simulink model "LateralControllerDIY"  (R2021a)
settings: Solver=VariableStepAuto  StartTime=0.0  StopTime=20  RelTol=1e-3
values from neighbouring files (symbols this model uses):
  ks = 0    [controller_setup.m]    (also in test.m)
  PredictionHorizon = 60    [controller_setup.m]
  Ts = 0.05    [controller_setup.m]    (also in test.m = 0.1)
  Vx = 15    [controller_setup.m]    (also in test.m)
libraries: simulink_extras x3, mpclib x1
(part 1 of 2)
settings Model: Creator=chnwa  LastModifiedBy=chnwa

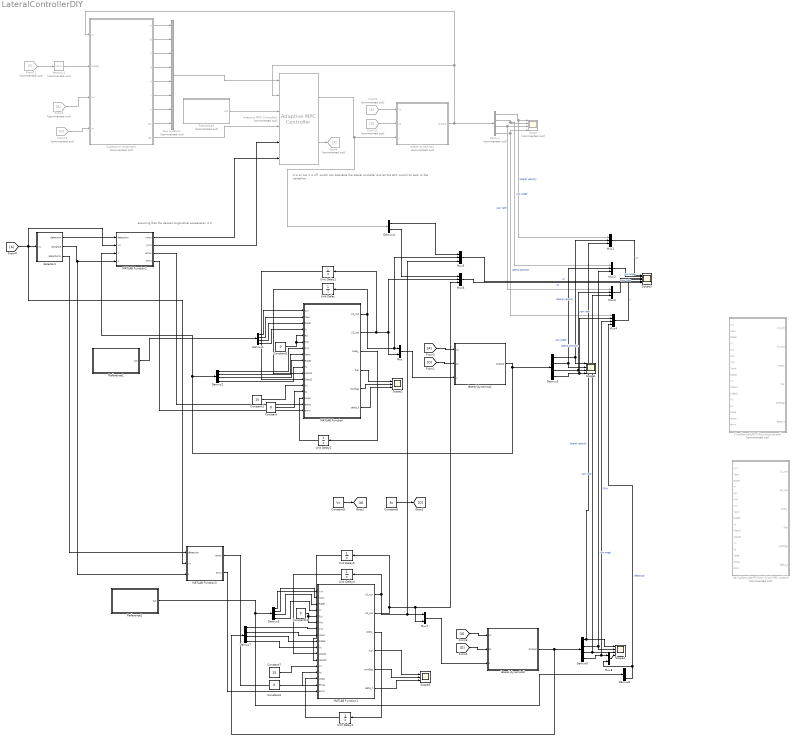
== system LateralControllerDIY ==
  note: assuming that the desired longitudinal acceleration is 0
  note: 0 is on but 1 is off. switch can disenable the lateral controller and let the ACC control its back to the centerline
  Adaptive MPC Controller1 : mpclib/Adaptive MPC Controller  Commented=on  SCDEnableBlockLinearizationSpecification=on  mpcobj=mpc007  enable_value=0  updateMPCinCallerWorkspace=on  md_inport=on  mv_inport=off  uref_inport=off  return_cost=off  return_mvseq=on  return_qpstatus=off  return_xseq=off  return_state=off  return_ovseq=off  state_inport=off  isltv_plant=on  umin_inport=off  umax_inport=off  ymin_inport=on  ymax_inport=on  cc_inport=off  ywt_inport=off  uwt_inport=off  duwt_inport=off  rhoeps_inport=off  pm_inport=off  MaximumP=10  HorizonChoice=FixedHorizon  BlockDataType=double  SampleTimeInherited=off  switch_inport=off
  Bus Creator1 : BusCreator  Commented=on  Inputs=8
  Constant{,2,4,10} (4 alike) : Constant  Value=0
  Constant1 : Constant  Value=15
  Constant5 : Constant  Value=Vx
  Constant6 : Constant  Value=ks
  Constant7 : Constant  Value=15
  Demux : Demux  Commented=on
  Demux{1..3,5..8} (7 alike) : Demux
  Demux4 : Demux  Outputs=2
  FixedSampleMPC(Non-Augmented) : MATLAB Function  Commented=on  TreatAsAtomicUnit=on
  From11 : From  Commented=on  GotoTag=F
  From12 : From  Commented=on  GotoTag=D
  From13 : From  Commented=on  GotoTag=D
  From2 : From  Commented=on
  From8 : From  Commented=on
  Goto6 : Goto  Commented=on  GotoTag=F
  MATLAB Function : MATLAB Function  TreatAsAtomicUnit=on
  MATLAB Function1 : MATLAB Function  TreatAsAtomicUnit=on
  MATLAB Function2 : MATLAB Function  TreatAsAtomicUnit=on
  MATLAB Function3 : MATLAB Function  TreatAsAtomicUnit=on
  Memory1 : Memory  Commented=on
  Mux : Mux  Inputs=2
  Mux{1..3,5..6} (5 alike) : Mux  Inputs=3
  Mux4 : Mux
  Mux7 : Mux  Inputs=2
  Mux8 : Mux  Inputs=2
  Reference1 : Subsystem  AncestorBlock=Meldas_library/Reference
  Reference2 : Subsystem  AncestorBlock=Meldas_library/Reference
  Reference3 : Subsystem  Commented=on  AncestorBlock=Meldas_library/Reference
  Scope : Scope  Commented=on  NumInputPorts=4
  Scope1 : Scope  NumInputPorts=4
  Scope2 : Scope  NumInputPorts=3
  Scope3 : Scope  NumInputPorts=6
  Scope4 : Scope  NumInputPorts=4
  Scope5 : Scope  NumInputPorts=3
  Successive Linearizer1 : MATLAB Function  Commented=on  TreatAsAtomicUnit=on
  Unit Delay{,1,4..5} (4 alike) : UnitDelay  SampleTime=-1  HasFrameUpgradeWarning=on
  Unit Delay2 : UnitDelay  InitialCondition=zeros(61,2)  SampleTime=-1  HasFrameUpgradeWarning=on
  Unit Delay3 : UnitDelay  InitialCondition=zeros(71,2)  SampleTime=-1  HasFrameUpgradeWarning=on
  VaringSampleMPC(Non-fixed MPC added) : MATLAB Function  Commented=on  TreatAsAtomicUnit=on
  detector1 : Subsystem
  lateral dynamics1 : Subsystem
  lateral dynamics2 : Subsystem  Commented=on
  lateral dynamics3 : Subsystem
  wires:
  Adaptive MPC Controller1/1 -> Demux4/1, lateral dynamics2/3(u)
  Constant6/1 -> [D]
  MATLAB Function2/2(ymin) -> Adaptive MPC Controller1/5
  Constant5/1 -> [A]
  Memory1/1 -> Successive Linearizer1/2(moves)
  From2/1 -> Successive Linearizer1/3(Vx)
  From8/1 -> lateral dynamics2/1(Vx)
  lateral dynamics2/1(Output) -> Demux/1, Successive Linearizer1/1(xk), Adaptive MPC Controller1/2
  From12/1 -> lateral dynamics2/2(ks)
  Successive Linearizer1/3(C) -> Bus Creator1/3
  Successive Linearizer1/5(U) -> Bus Creator1/5
  Successive Linearizer1/4(D) -> Bus Creator1/4
  Successive Linearizer1/2(B) -> Bus Creator1/2
  Bus Creator1/1 -> Adaptive MPC Controller1/1
  Successive Linearizer1/1(A) -> Bus Creator1/1
  Reference3/1(out) -> Adaptive MPC Controller1/3
  From13/1 -> Successive Linearizer1/4(ks)
  Successive Linearizer1/6(Y) -> Bus Creator1/6
  Successive Linearizer1/7(X) -> Bus Creator1/7
  detector1/2(distance) -> MATLAB Function3/3(s), MATLAB Function2/4(s)
  From11/1 -> Memory1/1
  MATLAB Function2/1(ymax) -> Adaptive MPC Controller1/6
  [A] -> MATLAB Function3/2(Vx), MATLAB Function2/2(Vx), detector1/1(Vx)
  Successive Linearizer1/8(DX) -> Bus Creator1/8
  Adaptive MPC Controller1/2 -> Goto6/1
  Successive Linearizer1/9(DK) -> Adaptive MPC Controller1/4
  Demux/1 -> Mux1/1, Scope/1  "lateral velocity"
  Demux/2 -> Mux2/1, Scope/2  "yaw angel"
  Demux/3 -> Mux3/1, Scope/3  "yaw rate"
  Demux/4 -> Mux4/1, Scope/4  "lateral position"
  MATLAB Function/1(U1_out) -> Mux5/2, Mux/1, Unit Delay/1
  Unit Delay/1 -> MATLAB Function/11(Ulast1)
  MATLAB Function/2(U2_out) -> Mux6/2, Mux/2, Unit Delay1/1
  Unit Delay1/1 -> MATLAB Function/12(Ulast2)
  MATLAB Function/3(Useq_) -> Unit Delay2/1
  Unit Delay2/1 -> MATLAB Function/15(Useq)
  Constant/1 -> MATLAB Function/14(ks)
  Constant1/1 -> MATLAB Function/13(Vx)
  Reference1/1(out) -> Demux1/1
  Demux1/1 -> MATLAB Function/1(Vyr)
  Demux1/2 -> MATLAB Function/2(Yawr)
  Demux1/3 -> MATLAB Function/3(Rater)
  Demux1/4 -> MATLAB Function/4(Yr)
  Constant2/1 -> MATLAB Function/5(Fyr), MATLAB Function/6(Mxr)
  [A] -> lateral dynamics1/1(Vx)
  [D] -> lateral dynamics1/2(ks)
  Mux/1 -> lateral dynamics1/3(u)
  Demux2/1 -> MATLAB Function/7(Vyc)
  Demux2/2 -> MATLAB Function/8(Yawc)
  Demux2/3 -> MATLAB Function/9(Ratec)
  Demux2/4 -> MATLAB Function/10(Yc)
  Demux3/2 -> Scope1/2, Mux2/2  "yaw angel"
  Demux3/3 -> Mux3/2, Scope1/3  "yaw rate"
  Demux3/1 -> Scope1/1, Mux1/2  "lateral velocity"
  lateral dynamics1/1(Output) -> MATLAB Function2/3(x), Demux2/1, Demux3/1
  Demux3/4 -> Mux4/2, Scope1/4  "lateral position"
  MATLAB Function/4(fval) -> Scope2/1
  MATLAB Function/5(exitflag) -> Scope2/2
  MATLAB Function/6(delta_t) -> Scope2/3
  Mux1/1 -> Scope3/1  "Vy"
  Mux2/1 -> Scope3/2  "yaw angle"
  Mux3/1 -> Scope3/3  "yaw rate"
  Mux4/1 -> Scope3/4  "Y"
  Demux4/1 -> Mux5/1
  Demux4/2 -> Mux6/1
  Mux5/1 -> Scope3/5  "u1"
  Mux6/1 -> Scope3/6  "u2"
  MATLAB Function1/1(U1_out) -> Unit Delay4/1, Mux5/3, Mux7/1
  Unit Delay4/1 -> MATLAB Function1/11(Ulast1)
  MATLAB Function1/2(U2_out) -> Mux6/3, Mux7/2, Unit Delay5/1
  Unit Delay5/1 -> MATLAB Function1/12(Ulast2)
  MATLAB Function1/3(Useq_) -> Unit Delay3/1
  Unit Delay3/1 -> MATLAB Function1/15(Useq)
  Constant7/1 -> MATLAB Function1/13(Vx)
  Constant4/1 -> MATLAB Function1/14(ks)
  Demux5/4 -> MATLAB Function1/4(Yr)
  Reference2/1(out) -> Demux8/1, Demux5/1
  Demux5/3 -> MATLAB Function1/3(Rater)
  Demux5/2 -> MATLAB Function1/2(Yawr)
  Demux5/1 -> MATLAB Function1/1(Vyr)
  Constant10/1 -> MATLAB Function1/5(Fyr), MATLAB Function1/6(Mxr)
  [A] -> lateral dynamics3/1(Vx)
  [D] -> lateral dynamics3/2(ks)
  Mux7/1 -> lateral dynamics3/3(u)
  Demux6/2 -> Mux2/3, Scope4/2  "yaw angel"
  Demux6/3 -> Scope4/3, Mux3/3  "yaw rate"
  Demux6/1 -> Mux1/3, Scope4/1  "lateral velocity"
  lateral dynamics3/1(Output) -> Demux7/1, Demux6/1
  Demux6/4 -> Mux4/3, Mux8/1  "FOH"
  Demux7/1 -> MATLAB Function1/7(Vyc)
  Demux7/2 -> MATLAB Function1/8(Yawc)
  Demux7/3 -> MATLAB Function1/9(Ratec)
  Demux7/4 -> MATLAB Function1/10(Yc)
  MATLAB Function1/4(fval) -> Scope5/1
  MATLAB Function1/6(delta_t) -> Scope5/3
  MATLAB Function1/5(exitflag) -> Scope5/2
  MATLAB Function2/3(emax) -> MATLAB Function/16(emax)
  MATLAB Function2/4(emin) -> MATLAB Function/17(emin)
  detector1/1(detection) -> MATLAB Function2/1(detection)
  Demux8/4 -> Mux4/4, Mux8/2  "reference"
  Mux8/1 -> Scope4/4
  detector1/3(detection1) -> MATLAB Function3/1(detection)
  MATLAB Function3/1(emax) -> MATLAB Function1/16(emax)
  MATLAB Function3/2(emin) -> MATLAB Function1/17(emin)

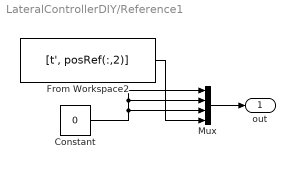
== system LateralControllerDIY/Reference1 ==
  Constant : Constant  Value=0
  From Workspace2 : FromWorkspace  VariableName=[t', posRef(:,2)]  SampleTime=0.1
  Mux : Mux
  out : Outport  VectorParamsAs1DForOutWhenUnconnected=off
  wires:
  From Workspace2/1 -> Mux/4
  Constant/1 -> Mux/3, Mux/2, Mux/1
  Mux/1 -> out/1

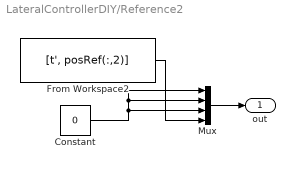
== system LateralControllerDIY/Reference2 ==
  Constant : Constant  Value=0
  From Workspace2 : FromWorkspace  VariableName=[t', posRef(:,2)]  SampleTime=0.1
  Mux : Mux
  out : Outport  VectorParamsAs1DForOutWhenUnconnected=off
  wires:
  From Workspace2/1 -> Mux/4
  Constant/1 -> Mux/3, Mux/2, Mux/1
  Mux/1 -> out/1

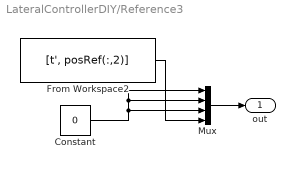
== system LateralControllerDIY/Reference3 ==
  Constant : Constant  Value=0
  From Workspace2 : FromWorkspace  VariableName=[t', posRef(:,2)]  SampleTime=0.1
  Mux : Mux
  out : Outport  VectorParamsAs1DForOutWhenUnconnected=off
  wires:
  From Workspace2/1 -> Mux/4
  Constant/1 -> Mux/3, Mux/2, Mux/1
  Mux/1 -> out/1

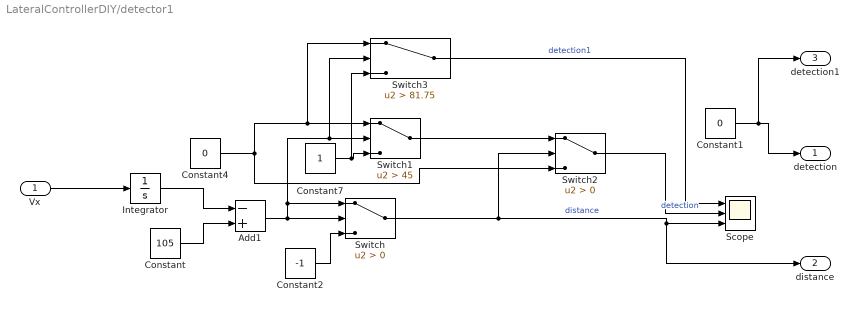
== system LateralControllerDIY/detector1 ==
  Vx : Inport
  Add1 : Sum  Inputs=-+
  Constant : Constant  Value=105
  Constant1 : Constant  Value=0
  Constant2 : Constant  Value=-1
  Constant4 : Constant  Value=0
  Constant7 : Constant
  Integrator : Integrator
  Scope : Scope  NumInputPorts=3
  Switch : Switch  Criteria=u2 > Threshold
  Switch1 : Switch  Criteria=u2 > Threshold  Threshold=45
  Switch2 : Switch  Criteria=u2 > Threshold
  Switch3 : Switch  Criteria=u2 > Threshold  Threshold=81.75
  detection : Outport
  distance : Outport  Port=2
  detection1 : Outport  Port=3
  wires:
  Constant2/1 -> Switch/3
  Constant4/1 -> Switch2/3, Switch3/1, Switch1/1
  Vx/1 -> Integrator/1
  Integrator/1 -> Add1/1
  Switch/1 -> Switch2/2, distance/1, Scope/3  "distance"
  Constant7/1 -> Switch3/3, Switch1/3
  Add1/1 -> Switch3/2, Switch1/2, Switch/1, Switch/2
  Switch1/1 -> Switch2/1
  Constant/1 -> Add1/2
  Switch2/1 -> Scope/2  "detection"
  Switch3/1 -> Scope/1  "detection1"
  Constant1/1 -> detection1/1, detection/1

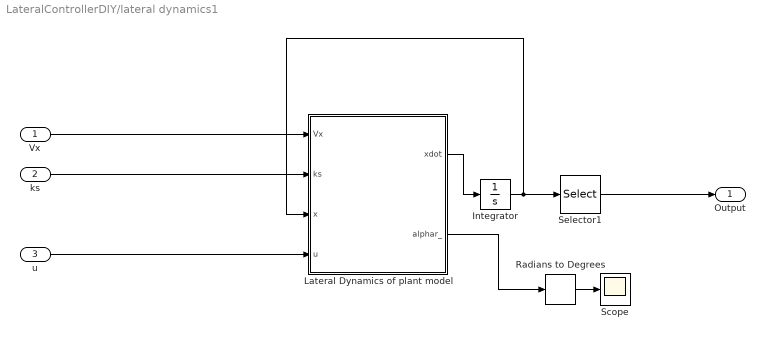
== system LateralControllerDIY/lateral dynamics1 ==
  Vx : Inport
  ks : Inport  Port=2
  u : Inport  Port=3
  Integrator : Integrator
  Lateral Dynamics of plant model : MATLAB Function  TreatAsAtomicUnit=on
  Radians to Degrees : simulink_extras/Transformations/Radians to Degrees
  Scope : Scope
  Selector1 : Selector  InputPortWidth=4  IndexOptions=Index vector (dialog)  Indices=[1 2 3 4]  OutputSizes=1
  Output : Outport
  wires:
  u/1 -> Lateral Dynamics of plant model/4(u)
  Lateral Dynamics of plant model/1(xdot) -> Integrator/1
  Integrator/1 -> Selector1/1, Lateral Dynamics of plant model/3(x)
  Selector1/1 -> Output/1
  ks/1 -> Lateral Dynamics of plant model/2(ks)
  Vx/1 -> Lateral Dynamics of plant model/1(Vx)
  Lateral Dynamics of plant model/2(alphar_) -> Radians to Degrees/1
  Radians to Degrees/1 -> Scope/1

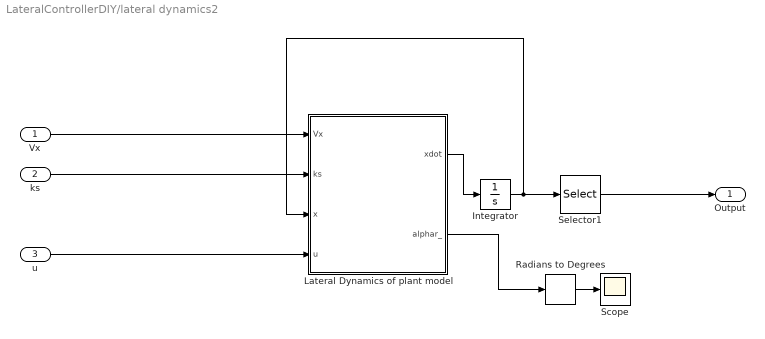
== system LateralControllerDIY/lateral dynamics2 ==
  Vx : Inport
  ks : Inport  Port=2
  u : Inport  Port=3
  Integrator : Integrator
  Lateral Dynamics of plant model : MATLAB Function  TreatAsAtomicUnit=on
  Radians to Degrees : simulink_extras/Transformations/Radians to Degrees
  Scope : Scope
  Selector1 : Selector  InputPortWidth=4  IndexOptions=Index vector (dialog)  Indices=[1 2 3 4]  OutputSizes=1
  Output : Outport
  wires:
  u/1 -> Lateral Dynamics of plant model/4(u)
  Lateral Dynamics of plant model/1(xdot) -> Integrator/1
  Integrator/1 -> Selector1/1, Lateral Dynamics of plant model/3(x)
  Selector1/1 -> Output/1
  ks/1 -> Lateral Dynamics of plant model/2(ks)
  Vx/1 -> Lateral Dynamics of plant model/1(Vx)
  Lateral Dynamics of plant model/2(alphar_) -> Radians to Degrees/1
  Radians to Degrees/1 -> Scope/1

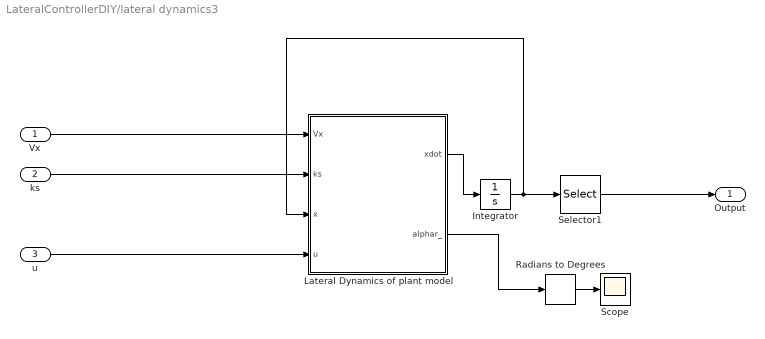
== system LateralControllerDIY/lateral dynamics3 ==
  Vx : Inport
  ks : Inport  Port=2
  u : Inport  Port=3
  Integrator : Integrator
  Lateral Dynamics of plant model : MATLAB Function  TreatAsAtomicUnit=on
  Radians to Degrees : simulink_extras/Transformations/Radians to Degrees
  Scope : Scope
  Selector1 : Selector  InputPortWidth=4  IndexOptions=Index vector (dialog)  Indices=[1 2 3 4]  OutputSizes=1
  Output : Outport
  wires:
  u/1 -> Lateral Dynamics of plant model/4(u)
  Lateral Dynamics of plant model/1(xdot) -> Integrator/1
  Integrator/1 -> Selector1/1, Lateral Dynamics of plant model/3(x)
  Selector1/1 -> Output/1
  ks/1 -> Lateral Dynamics of plant model/2(ks)
  Vx/1 -> Lateral Dynamics of plant model/1(Vx)
  Lateral Dynamics of plant model/2(alphar_) -> Radians to Degrees/1
  Radians to Degrees/1 -> Scope/1

== matlab function LateralControllerDIY/Successive Linearizer1 ==
  data: A output size=[4,4,PredictionHorizon+1]; xk input size=[4,1]; moves input; B output size=[4,6,PredictionHorizon+1]; C output size=[4,4,PredictionHorizon+1]; D output size=[4,6,PredictionHorizon+1]; U output size=[6,1,PredictionHorizon+1]; Y output size=[4,1,PredictionHorizon+1]; X output size=[4,1,PredictionHorizon+1]; DX output size=[4,1,PredictionHorizon+1]; Vx input size=1; ks input; PredictionHorizon parameter size=1; DK output; Ts parameter size=1
function [A,B,C,D,U,Y,X,DX,DK] = fcn(xk,moves,Vx,ks, PredictionHorizon, Ts)
%sucessive updates the LTI plant model required by adaptive MPC controller
% LTV MPC requires p+1 linearizations from k to k+p
Steps = PredictionHorizon + 1; % having the number of Steps models
% Initialize outputs
A = zeros(4,4,Steps);
B = zeros(4,6,Steps);
C = zeros(4,4,Steps);
D = zeros(4,6,Steps);
U = zeros(6,1,Steps);
Y = zeros(4,1,Steps);
X = zeros(4,1,Steps);
DX = zeros(4,1,Steps);
DK = zeros(Steps,4); % the constant matrix in the model considered as measured disturbance

% Obtain time varying linear models via successive linearization
for ct = 1:Steps
    % since we don't have u(k) ... u(k+p) at the time of linearization,
    % previous optimal sequence u(k-1) ... u(k+p-1) is used instead.
    if ct>length(moves)
        uk = moves(Steps,:);
    else
        uk = moves(ct,:);
    end
    uk = uk';
    % analytical linearization (continuous time)
    [Ac, Bc, Cc, Dc, dc] = LateralDynamicsCT(Vx,ks,xk); % acquiring new characteristic matrix
    % convert A and B matrices from continuous time to discrete time
    % augmenting the model to be in the form of dotX=A*x+B*u while u=[u;dc]
    Aca = Ac;
    Bca = [Bc eye(4)];
    M = expm([[Aca Bca zeros(4,1)]*Ts;zeros(7,11)]);
    Ak = M(1:4,1:4);    %the discrete matrix A for augmented model
    Bk = M(1:4,5:10);   %the discrete matrix B for augmented model
    %store the state space matrix for ct time step
    A(:,:,ct) = Ak;
    B(:,:,ct) = Bk;
    C(:,:,ct) = Cc;
    D(:,:,ct) = [Dc,zeros(4,4)];  % always be zeros(4,6) in fact
    U(:,:,ct) = [uk;dc];          % measured disturbance dc is input as well
    Y(:,:,ct) = xk;               % output is all of the four states
    X(:,:,ct) = xk;               % four states
    DX(:,:,ct) = Ak*xk+Bk*[uk;dc]-xk;%the states increment
    DK(ct,:) = dc';               % disturbance in this step
    % next prediction step
    xk = DX(:,:,ct)+xk;           %update the states
end

%%%unrelated stuff
% ct= LTVu15_dist_Ts01.Model.Plant;
% dt = c2d(ct,Ts);
% LTVu15_dist_Ts01.Model.Plant = dt;

== matlab function LateralControllerDIY/lateral dynamics2/Lateral Dynamics of plant model ==
  data: Vx input; ks input; x input; u input; xdot output; alphar_ output
function [xdot,alphar_] = fcn(Vx,ks, x, u)

%Plant Model parameters
m = 2272;   %mass
Iz = 4600;  %rotational inertia
lf = 1.11;  % distance from front axle to the mass center
lr = 1.67;  % distance from rear axle to the mass center
C_a = 1.822e5; % rear cornering stifness 

%Enviroment parameters
miu = 0.7; %frction cooeficient 0.7 for dry road and 0.4 for wet
g = 9.81; % gravity

Fz = m*g*lf/(lf+lr); % the load that beared by the rear tire

%calculate alpha
Vy = x(1); %lateral velocity
r = x(2);  %yaw rate
alphar_ = Vy/Vx-lr*r/Vx;   %calculate linearzing point

%tire model
threshold = atan(3*miu*Fz/C_a);
if abs(alphar_)<threshold
    Fyr_ = -C_a*tan(alphar_)+C_a^2/(3*miu*Fz)*abs(tan(alphar_))*tan(alphar_)-C_a^3/(27*miu^2*Fz^2)*tan(alphar_)^3;
    if alphar_>= 0
        Cr_ = -C_a*sec(alphar_)^2+C_a^2/(3*miu*Fz)*(2*sec(alphar_)^2*tan(alphar_))-C_a^3/(27*miu^2*Fz^2)*(3*tan(alphar_)^2*sec(alphar_)^2);
    else
        Cr_ = -C_a*sec(alphar_)^2-C_a^2/(3*miu*Fz)*(2*sec(alphar_)^2*tan(alphar_))-C_a^3/(27*miu^2*Fz^2)*(3*tan(alphar_)^2*sec(alphar_)^2);
    end
else
    Fyr_ = -miu*Fz*sign(alphar_);
    Cr_ = 0;
end

%Continuous-time model
Ac = [Cr_/(m*Vx) -lr*Cr_/(m*Vx)-Vx 0 0;
    -lr*Cr_/(Iz*Vx) lr^2*Cr_/(Iz*Vx) 0 0;
    0 1 0 0;
    1 0 Vx 0];
Bc = [1/m 0;
    lf/Iz 1/Iz;
    0 0;
    0 0];
dcc = [(Fyr_-Cr_*alphar_)/m;
    -lr*(Fyr_-Cr_*alphar_)/Iz;
    -Vx*ks;
    0];

% Cc =eye(4);
% Dc =zeros(4,2);
xdot = Ac*x + Bc*u +dcc;
% y = C*x + D*u;

== matlab function LateralControllerDIY/lateral dynamics3/Lateral Dynamics of plant model ==
  data: Vx input; ks input; x input; u input; xdot output; alphar_ output
function [xdot,alphar_] = fcn(Vx,ks, x, u)

%Plant Model parameters
m = 2272;   %mass
Iz = 4600;  %rotational inertia
lf = 1.11;  % distance from front axle to the mass center
lr = 1.67;  % distance from rear axle to the mass center
C_a = 1.822e5; % rear cornering stifness 

%Enviroment parameters
miu = 0.7; %frction cooeficient 0.7 for dry road and 0.4 for wet
g = 9.81; % gravity

Fz = m*g*lf/(lf+lr); % the load that beared by the rear tire

%calculate alpha
Vy = x(1); %lateral velocity
r = x(2);  %yaw rate
alphar_ = Vy/Vx-lr*r/Vx;   %calculate linearzing point

%tire model
threshold = atan(3*miu*Fz/C_a);
if abs(alphar_)<threshold
    Fyr_ = -C_a*tan(alphar_)+C_a^2/(3*miu*Fz)*abs(tan(alphar_))*tan(alphar_)-C_a^3/(27*miu^2*Fz^2)*tan(alphar_)^3;
    if alphar_>= 0
        Cr_ = -C_a*sec(alphar_)^2+C_a^2/(3*miu*Fz)*(2*sec(alphar_)^2*tan(alphar_))-C_a^3/(27*miu^2*Fz^2)*(3*tan(alphar_)^2*sec(alphar_)^2);
    else
        Cr_ = -C_a*sec(alphar_)^2-C_a^2/(3*miu*Fz)*(2*sec(alphar_)^2*tan(alphar_))-C_a^3/(27*miu^2*Fz^2)*(3*tan(alphar_)^2*sec(alphar_)^2);
    end
else
    Fyr_ = -miu*Fz*sign(alphar_);
    Cr_ = 0;
end

%Continuous-time model
Ac = [Cr_/(m*Vx) -lr*Cr_/(m*Vx)-Vx 0 0;
    -lr*Cr_/(Iz*Vx) lr^2*Cr_/(Iz*Vx) 0 0;
    0 1 0 0;
    1 0 Vx 0];
Bc = [1/m 0;
    lf/Iz 1/Iz;
    0 0;
    0 0];
dcc = [(Fyr_-Cr_*alphar_)/m;
    -lr*(Fyr_-Cr_*alphar_)/Iz;
    -Vx*ks;
    0];

% Cc =eye(4);
% Dc =zeros(4,2);
xdot = Ac*x + Bc*u +dcc;
% y = C*x + D*u;

== matlab function LateralControllerDIY/VaringSampleMPC(Non-fixed MPC added) ==
  data: Vyr input; U1_out output; Yawr input; Rater input; Yr input; Fyr input; Mxr input; Vyc input; Yawc input; Ratec input; Yc input; Ulast1 input; Ulast2 input; Vx input; ks input; Useq input; U2_out output; Useq_ output; fval output; exitflag output; delta_t output; emax input; emin input
function [U1_out,U2_out,Useq_,fval,exitflag,delta_t] = fcn(Vyr,Yawr,Rater,Yr, Fyr,Mxr,Vyc,Yawc,Ratec,Yc,Ulast1,Ulast2,Vx,ks,Useq,emax,emin)
%Vyr lateral velocity, Yawr yaw angle, Rater yaw rate, Yr lateral position
%Fyr lateral force in front tyre,Mxr moment generated by longitudinal force
%'r'means reference ||  'c'means current
% Ulast1,Ulast2 are u(k-1), Ucrnt1,Ucrnt2 are u(k) calculated from last
% control period
    if Vx<0.1
        Vx=0.001;%make sure many expressions' denominator isn't 0
    end
    lr=1.67;
    threshold=0.1022;
    miu=0.7;
    rmax=9.81*miu/Vx;
%% Initilization    
    tstart=tic;%timing on
    
    Nx=4;%number of state
    Nu=2;%number of control(FOH should be twice)
    Np=30;%prediction horizon
    %N1 cannot be equal to N2
    N1=15;
    N2=5;
%     N3=20;
    Nc=1;%control horizon

    %reference
    r=zeros(Nx,1);%state reference
    r(1)=Vyr;
    r(2)=Yawr;
    r(3)=Rater;
    r(4)=Yr;    
    ur1=Fyr;
    ur2=Mxr;%control reference
    
    %states
    x=zeros(Nx,1);%state reference
    x(1)=Vyc;
    x(2)=Yawc;
    x(3)=Ratec;
    x(4)=Yc;   
    
    %control
    u=zeros(Nu,1);%state reference
    u(1)=Ulast1;
    u(2)=Ulast2;
    
    %get augmented states
    kesi=zeros(Nx+Nu,1);%[X;U]
    kesi(1)=x(1)-r(1);
    kesi(2)=x(2)-r(2);
    kesi(3)=x(3)-r(3);
    kesi(4)=x(4)-r(4);
    kesi(5)=u(1)-ur1;
    kesi(6)=u(2)-ur2;
    
%% Modellng->Discretization->prediction->quadratic programming
    %sample time 
    Ts1=0.05;
    Ts2=0.05;
    %Modelling&Linearization&Discretization
    steps=Np+1;
    A = zeros(Nx+Nu,Nx+Nu,steps);
    B = zeros(Nx+Nu,Nu*2,steps);
    Dc = zeros(Nx+Nu,1,steps);
    C=[1 0 0 0 0 0;0 1 0 0 0 0;0 0 1 0 0 0;0 0 0 1 0 0];
    
    for ct = 1:steps
        if ct<=N1
            Ts=Ts1;
        elseif ct<=N1+N2
            Ts=Ts1+(Ts2-Ts1)*(ct-N1)/(N2-N1);
        else
            Ts=Ts2;
        end    
        uk = Useq(ct,:);
        if ct == steps
            uk1 = Useq(ct,:);
        else
            uk1= Useq(ct+1,:);
        end
        uk=uk';
        uk1=uk1';
        [Ad, Bd1,Bd2, DK, delta_x] = GetDynamicsFOH(Vx,ks,x,uk,uk1,Ts);
        A(:,:,ct)=[Ad Bd1+Bd2;zeros(Nu,Nx) eye(Nu)];        
        B(:,:,ct)=[Bd1+Bd2 Bd2;eye(Nu) zeros(Nu,Nu)];
        Dc(:,:,ct)=[DK;0;0];
        x=x+delta_x;    
    end
    %construct important matrix
    %Y=PHI*kesi+THETA*delta_U+OMEGA*D
    coder.varsize('PHI',[Np*Nx,Nx+Nu]);
    coder.varsize('THETA',[Np*Nx,2*Nu]);
    coder.varsize('D',[Np*(Nx+Nu),1]);
    coder.varsize('DD',[Np*Nx,1]);
    PHI=[];
    THETA=zeros(Np*Nx,2*Nu);
    D=[];
    product=eye(6);
    for j=1:Np
        product=A(:,:,j)*product;
        PHI=[PHI;C*product];
        D=[D;Dc(:,:,j)];
    end
    for k=1:Nc
        product1=eye(6);
        for j=k:Np
            THETA(4*j-3:4*j,4*k-3:4*k)=C*product1*B(:,:,Nc);
            product1=A(:,:,j+1)*product1;
        end
    end
    coder.varsize('OMEGA',[Nx*Np,(Nx+Nu)*Np]);
    OMEGA=zeros(Nx*Np,(Nx+Nu)*Np);
    for i=1:Np
        product2=A(:,:,i+1);
        for j=i:Np-1
            if i==j
                OMEGA(4*i-3:4*i,6*i-5:6*i)=C*eye(6);
            end
            OMEGA(4*j+1:4*j+4,6*j+1:6*j+6)=C*product2;
            product2=A(:,:,j+2)*product2;
        end
    end
    DD=OMEGA*D;        
    Sigma=repmat([1 0 1 0;0 1 0 1],Np,1);
    Sigma(1:2,1:4)=[1 0 0 0;0 1 0 0];
    UT=kron(ones(Np,1),[u(1);u(2)]); %=repmat([u(1);u(2);u(3);u(4)],Np,1) %(Nu*Np,1)
    error=PHI*kesi;%(Nx*Np,Nx+Nu)*(Nu+Nx,1)
    Q=kron(eye(Np,Np),diag([0 0 100 4]));    
    R=kron(eye(Np,Np),diag([0 4e-5]));    
    P=diag([3e-5 8e-5 3e-5 8e-5]);%deltaU（k+1）是否应该与deltaU（k）一样呢
    rou1=3e3;    
    rou2=5e4;
    H=2*[THETA'*Q*THETA+Sigma'*R*Sigma+P zeros(4,2);zeros(1,4) rou1 0;zeros(1,4) 0 rou2];%是否要乘2？要
    f=[2*(error'*Q*THETA+(OMEGA*D)'*Q*THETA+UT'*R*Sigma),0,0];%是否要转置？好像无所谓
   %% constraints
    %inequation
    A_I=[1 0 0 0;0 1 0 0;1 0 1 0;0 1 0 1]; 
    Ut=kron(ones(2,1),[Ulast1;Ulast2]);%control in last control step
    umin=[-1e4; -1e3];
    umax=[1e4; 1e3];
    Umin=kron(ones(2,1),umin);
    Umax=kron(ones(2,1),umax);
    coder.varsize('A_cons',[Np*6+8,6]);
    coder.varsize('b_cons',[Np*6+8,1]);
    A_cons=[A_I zeros(4,2);-A_I zeros(4,2)];
    b_cons=[Umax-Ut;-Umin+Ut];
    %add handling envelop constriants & environment envolop
    gamas=[1 -lr 0 0;-1 lr 0 0;0 1 0 0;0 -1 0 0];
    gamae=[0 0 0 1;0 0 0 -1];
    Gs=[Vx*threshold;Vx*threshold;rmax;rmax];
    for i=1:Np
        A_cons=[A_cons;[gamas*THETA(4*i-3:4*i,:) -ones(4,1) zeros(4,1)];[gamae*THETA(4*i-3:4*i,:) zeros(2,1) -ones(2,1)]];
        b_cons=[b_cons;[Gs-gamas*(PHI(4*i-3:4*i,:)*kesi-DD(4*i-3:4*i,:))];[emax(i);-emin(i)]-gamae*(PHI(4*i-3:4*i,:)*kesi-DD(4*i-3:4*i,:))];
    end
    
    %upper and lower boundary
    delta_umin=[-1e4;-1e3];
    delta_umax=[1e4;1e3];
    M1=10; %related to slack variable
    M2=10; %related to slack variable
    delta_Umin=kron(ones(2,1),delta_umin);
    delta_Umax=kron(ones(2,1),delta_umax);
    lb=[delta_Umin;0;0];
    ub=[delta_Umax;M1;M2];  
   %% solve quadratic programming
    opts = optimoptions('quadprog','Algorithm','active-set');
    x_start=zeros(Nu*2+2,1);%+2 corresponds to slack variables
    [X,fval,exitflag]=quadprog(H,f',A_cons,b_cons,[],[],lb,ub,x_start,opts);
    
   %% calculate control signal
    U1=kesi(5)+X(1);%The output error at the previous time plus the optimization result to get the error at this time
    U2=kesi(6)+X(2);%The output error at the previous time plus the optimization result to get the error at this time
    U1_out=U1+ur1;%Error plus reference value to get final output value    
    U2_out=U2+ur2;
    Useq_=[U1_out U2_out; repmat([U1_out+X(3) U2_out+X(4)],Np,1)];
    delta_t=toc(tstart);%timing off
end

% function [A, B, DK, delta_x] = GetDynamicsZOH(Vx,ks,x,u,Ts)
% 
% %Plant Model parameters
% m = 2272;   %mass
% Iz = 4600;  %rotational inertia
% lf = 1.11;  % distance from front axle to the mass center
% lr = 1.67;  % distance from rear axle to the mass center
% C_a = 1.822e5; % rear cornering stiffness 
% 
% %Enviroment parameters
% miu = 0.7; %frction cooeficient 0.7 for dry road and 0.4 for wet
% g = 9.81; % gravity
% 
% Fz = m*g*lf/(lf+lr); % the load that beared by the rear tire
% 
% %calculate alpha
% Vy = x(1); %lateral velocity
% r = x(2);  %yaw rate
% alphar_ = Vy/Vx-lr*r/Vx;   %calculate linearzing point
% 
% %tire model
% threshold = atan(3*miu*Fz/C_a);     % threshold for the tire linear region
% if abs(alphar_)<threshold
%     %the rear lateral force value (f(x0)) at the linearzing point
%     Fyr_ = -C_a*tan(alphar_)+C_a^2/(3*miu*Fz)*abs(tan(alphar_))*tan(alphar_)-C_a^3/(27*miu^2*Fz^2)*tan(alphar_)^3;
%     
%     %the slope of linearized model (f‘(x0))
%     if alphar_>= 0
%         Cr_ = -C_a*sec(alphar_)^2+C_a^2/(3*miu*Fz)*(2*sec(alphar_)^2*tan(alphar_))-C_a^3/(27*miu^2*Fz^2)*(3*tan(alphar_)^2*sec(alphar_)^2);
%     else
%         Cr_ = -C_a*sec(alphar_)^2-C_a^2/(3*miu*Fz)*(2*sec(alphar_)^2*tan(alphar_))-C_a^3/(27*miu^2*Fz^2)*(3*tan(alphar_)^2*sec(alphar_)^2);
%     end
% else
%     
%     %the saturation region of tire model
%     Fyr_ = -miu*Fz*sign(alphar_);
%     Cr_ = 0;
% end
% 
% %Continuous-time model
% Ac = [Cr_/(m*Vx) -lr*Cr_/(m*Vx)-Vx 0 0;
%     -lr*Cr_/(Iz*Vx) lr^2*Cr_/(Iz*Vx) 0 0;
%     0 1 0 0;
%     1 0 Vx 0];
% Bc = [1/m 0;
%     lf/Iz 1/Iz;
%     0 0;
%     0 0];
% dcc = [(Fyr_-Cr_*alphar_)/m;
%     -lr*(Fyr_-Cr_*alphar_)/Iz;
%     -Vx*ks;
%     0];
% 
% G=[Ac Bc dcc;zeros(3,7)];
% M=expm(G*Ts);
% A=M(1:4,1:4);
% B=M(1:4,5:6);
% DK=M(1:4,7);
% delta_x=A*x+B*u+DK-x;
% end

function [A, B1, B2, DK, delta_x] = GetDynamicsFOH(Vx,ks,x,uk,uk1,Ts)

%Plant Model parameters
m = 2272;   %mass
Iz = 4600;  %rotational inertia
lf = 1.11;  % distance from front axle to the mass center
lr = 1.67;  % distance from rear axle to the mass center
C_a = 1.822e5; % rear cornering stiffness 

%Enviroment parameters
miu = 0.7; %frction cooeficient 0.7 for dry road and 0.4 for wet
g = 9.81; % gravity

Fz = m*g*lf/(lf+lr); % the load that beared by the rear tire

%calculate alpha
Vy = x(1); %lateral velocity
r = x(2);  %yaw rate
alphar_ = Vy/Vx-lr*r/Vx;   %calculate linearzing point

%tire model
threshold = atan(3*miu*Fz/C_a);     % threshold for the tire linear region
if abs(alphar_)<threshold
    %the rear lateral force value (f(x0)) at the linearzing point
    Fyr_ = -C_a*tan(alphar_)+C_a^2/(3*miu*Fz)*abs(tan(alphar_))*tan(alphar_)-C_a^3/(27*miu^2*Fz^2)*tan(alphar_)^3;
    
    %the slope of linearized model (f‘(x0))
    if alphar_>= 0
        Cr_ = -C_a*sec(alphar_)^2+C_a^2/(3*miu*Fz)*(2*sec(alphar_)^2*tan(alphar_))-C_a^3/(27*miu^2*Fz^2)*(3*tan(alphar_)^2*sec(alphar_)^2);
    else
        Cr_ = -C_a*sec(alphar_)^2-C_a^2/(3*miu*Fz)*(2*sec(alphar_)^2*tan(alphar_))-C_a^3/(27*miu^2*Fz^2)*(3*tan(alphar_)^2*sec(alphar_)^2);
    end
else
    
    %the saturation region of tire model
    Fyr_ = -miu*Fz*sign(alphar_);
    Cr_ = 0;
end

%Continuous-time model
Ac = [Cr_/(m*Vx) -lr*Cr_/(m*Vx)-Vx 0 0;
    -lr*Cr_/(Iz*Vx) lr^2*Cr_/(Iz*Vx) 0 0;
    0 1 0 0;
    1 0 Vx 0];
Bc = [1/m 0;
    lf/Iz 1/Iz;
    0 0;
    0 0];
dcc = [(Fyr_-Cr_*alphar_)/m;
    -lr*(Fyr_-Cr_*alphar_)/Iz;
    -Vx*ks;
    0];

LAMDA=[Ac Bc dcc zeros(4,3);zeros(3,7) 1/Ts*eye(3);zeros(3,10)];
M=expm(LAMDA*Ts);
A=M(1:4,1:4);
PHI1=M(1:4,5:7);
PHI2=M(1:4,8:10);
B1=(PHI1-PHI2)*[eye(2);zeros(1,2)];
B2=PHI2*[eye(2);zeros(1,2)];
DK=PHI1*[0;0;1];
delta_x=A*x+B1*uk+B2*uk1+DK-x;
end

== matlab function LateralControllerDIY/FixedSampleMPC(Non-Augmented) ==
  data: Vyr input; U1_out output; Yawr input; Rater input; Yr input; Fyr input; Mxr input; Vyc input; Yawc input; Ratec input; Yc input; Ulast1 input; Ulast2 input; Vx input; ks input; Useq input; U2_out output; Useq_ output; fval output; exitflag output; delta_t output; emax input; emin input
function [U1_out,U2_out,Useq_,fval,exitflag,delta_t] = fcn(Vyr,Yawr,Rater,Yr, Fyr,Mxr,Vyc,Yawc,Ratec,Yc,Ulast1,Ulast2,Vx,ks,Useq,emax,emin)
%Vyr lateral velocity, Yawr yaw angle, Rater yaw rate, Yr lateral position
%Fyr lateral force in front tyre,Mxr moment generated by longitudinal force
%'r'means reference ||  'c'means current
    if Vx<0.1
        Vx=0.001;%make sure many expressions' denominator isn't 0
    end
    lr=1.67;
    threshold=0.1022;
    miu=0.7;
    rmax=9.81*miu/Vx;
%% Initilization    
    tstart=tic;%timing on
    
    Nx=4;%number of state
    Nu=2;%number of control
    Np=30;%prediction horizon
    Nc=1;%control horizon

    %reference
    r=zeros(Nx,1);%state reference
    r(1)=Vyr;
    r(2)=Yawr;
    r(3)=Rater;
    r(4)=Yr;    
    ur1=Fyr;
    ur2=Mxr;%control reference
    
    %states
    x=zeros(Nx,1);%state reference
    x(1)=Vyc;
    x(2)=Yawc;
    x(3)=Ratec;
    x(4)=Yc;   
    
    %control
    u=zeros(Nu,1);%state reference
    u(1)=Ulast1;
    u(2)=Ulast2;
    
    %get augmented states
    kesi=zeros(Nx+Nu,1);%[X;U]
    kesi(1)=x(1)-r(1);
    kesi(2)=x(2)-r(2);
    kesi(3)=x(3)-r(3);
    kesi(4)=x(4)-r(4);
    kesi(5)=u(1)-ur1;
    kesi(6)=u(2)-ur2;
    
    Ts=0.05;%sample time
    
%% Modellng->Discretization->prediction->quadratic programming
    %Modelling&Linearization&Discretization
    steps=Np+1;
    A = zeros(Nx+Nu,Nx+Nu,steps);
    B = zeros(Nx+Nu,Nu,steps);
    Dc = zeros(Nx+Nu,1,steps);
    C=[1 0 0 0 0 0;0 1 0 0 0 0;0 0 1 0 0 0;0 0 0 1 0 0];
    
    for ct = 1:steps
        if ct>length(Useq)
            uk = Useq(Np,:);
        else
            uk = Useq(ct,:);
        end
        uk=uk';
        [Ad, Bd, DK, delta_x] = GetDynamics(Vx,ks,x,uk,Ts);
        A(:,:,ct)=[Ad,Bd;zeros(Nu,Nx),eye(Nu)];        
        B(:,:,ct)=[Bd;eye(Nu)];
        Dc(:,:,ct)=[DK;0;0];
        x=x+delta_x;    
    end
    %construct important matrix
    %Y=PHI*kesi+THETA*delta_U+OMEGA*D
    coder.varsize('PHI',[Np*Nx,Nx+Nu]);
    coder.varsize('THETA',[Np*Nx,Nc*Nu]);
    coder.varsize('D',[Np*(Nx+Nu),1]);
    coder.varsize('DD',[Np*Nx,1]);
    PHI=[];
    THETA=[];
    D=[];
    DD=[];
    product=eye(6);
    for j=1:Np
        product=A(:,:,j)*product;
        PHI=[PHI;C*product];
        D=[D;Dc(:,:,j)];
    end
    for k=1:Nc
        product1=eye(6);
        for j=1:Np
            THETA=[THETA;C*product1*B(:,:,k)];
            product1=A(:,:,j+1)*product1;
        end
    end
    coder.varsize('OMEGA',[Nx*Np,(Nx+Nu)*Np]);
    OMEGA=zeros(Nx*Np,(Nx+Nu)*Np);
    for i=1:Np
        product2=A(:,:,i+1);
        for j=i:Np-1
            if i==j
                OMEGA(4*i-3:4*i,6*i-5:6*i)=C*eye(6);
            end
            OMEGA(4*j+1:4*j+4,6*j+1:6*j+6)=C*product2;
            product2=A(:,:,j+2)*product2;
        end
    end
    DD=OMEGA*D;        
    Sigma=zeros(Np,Nc);
    for p=1:Np%define a lower triangular matrix
        for q=1:1:Nc
            if q<=p 
                Sigma(p,q)=1;
            else 
                Sigma(p,q)=0;
            end
        end 
    end 
    UT=kron(ones(Np,1),[u(1);u(2)]);
    Sigma=kron(Sigma,eye(Nu));
    error=PHI*kesi;
    Q=kron(eye(Np,Np),diag([0 0 100 4]));    
    R=kron(eye(Np,Np),diag([0 4e-5]));    
    P=diag([3e-5 8e-5]);
    rou1=3e3;    
    rou2=5e4;
    H=2*[THETA'*Q*THETA+Sigma'*R*Sigma+P zeros(2,2);0 0 rou1 0;0 0 0 rou2];%是否要乘2？要
    f=[2*(error'*Q*THETA+(OMEGA*D)'*Q*THETA+UT'*R*Sigma),0,0];%是否要转置？好像无所谓
   %% constraints
    %inequation
    A_t=zeros(Nc,Nc);
    for p=1:1:Nc%define a lower triangular matrix
        for q=1:1:Nc
            if q<=p 
                A_t(p,q)=1;
            else 
                A_t(p,q)=0;
            end
        end 
    end 
    A_I=kron(A_t,eye(Nu)); 
    Ut=kron(ones(Nc,1),[Ulast1;Ulast2]);%control in last control step
    umin=[-1e4; -1e3];
    umax=[1e4; 1e3];
    Umin=kron(ones(Nc,1),umin);
    Umax=kron(ones(Nc,1),umax);
    coder.varsize('A_cons',[Np*6+4,4]);
    coder.varsize('b_cons',[Np*6+4,1]);
    A_cons=[A_I zeros(Nu*Nc,2);-A_I zeros(Nu*Nc,2)];
    b_cons=[Umax-Ut;-Umin+Ut];
    %add handling envelop constriants & environment envolop
    gamas=[1 -lr 0 0;-1 lr 0 0;0 1 0 0;0 -1 0 0];
    gamae=[0 0 0 1;0 0 0 -1];
    Gs=[Vx*threshold;Vx*threshold;rmax;rmax];
    for i=1:Np
        A_cons=[A_cons;[gamas*THETA(4*i-3:4*i,:) -ones(4,1) zeros(4,1)];[gamae*THETA(4*i-3:4*i,:) zeros(2,1) -ones(2,1)]];
        b_cons=[b_cons;[Gs-gamas*(PHI(4*i-3:4*i,:)*kesi-DD(4*i-3:4*i,:))];[emax(i);-emin(i)]-gamae*(PHI(4*i-3:4*i,:)*kesi-DD(4*i-3:4*i,:))];
    end
    
    %upper and lower boundary
    delta_umin=[-1e4;-1e3];
    delta_umax=[1e4;1e3];
    M1=10; %related to slack variable
    M2=10; %related to slack variable
    delta_Umin=kron(ones(Nc,1),delta_umin);
    delta_Umax=kron(ones(Nc,1),delta_umax);
    lb=[delta_Umin;0;0];
    ub=[delta_Umax;M1;M2];  
   %% solve quadratic programming
    opts = optimoptions('quadprog','Algorithm','active-set');
    x_start=zeros(Nu*Nc+2,1);%+2 corresponds to slack variables
    [X,fval,exitflag]=quadprog(H,f',A_cons,b_cons,[],[],lb,ub,x_start,opts);
    
   %% calculate control signal
    U1=kesi(5)+X(1);%The output error at the previous time plus the optimization result to get the error at this time
    U2=kesi(6)+X(2);%The output error at the previous time plus the optimization result to get the error at this time
    U1_out=U1+ur1;%Error plus reference value to get final output value    
    U2_out=U2+ur2;
    Useq_=repmat([U1,U2],Np+1,1); %adaptive MPC block's method
%     Useq_=[[U1,U2];repmat(zeros(1,2),Np,1)]; %this may make more sense
    delta_t=toc(tstart);%timing off
end

function [A, B, DK, delta_x] = GetDynamics(Vx,ks,x,u,Ts)

%Plant Model parameters
m = 2272;   %mass
Iz = 4600;  %rotational inertia
lf = 1.11;  % distance from front axle to the mass center
lr = 1.67;  % distance from rear axle to the mass center
C_a = 1.822e5; % rear cornering stiffness 

%Enviroment parameters
miu = 0.7; %frction cooeficient 0.7 for dry road and 0.4 for wet
g = 9.81; % gravity

Fz = m*g*lf/(lf+lr); % the load that beared by the rear tire

%calculate alpha
Vy = x(1); %lateral velocity
r = x(2);  %yaw rate
alphar_ = Vy/Vx-lr*r/Vx;   %calculate linearzing point

%tire model
threshold = atan(3*miu*Fz/C_a);     % threshold for the tire linear region
if abs(alphar_)<threshold
    %the rear lateral force value (f(x0)) at the linearzing point
    Fyr_ = -C_a*tan(alphar_)+C_a^2/(3*miu*Fz)*abs(tan(alphar_))*tan(alphar_)-C_a^3/(27*miu^2*Fz^2)*tan(alphar_)^3;
    
    %the slope of linearized model (f‘(x0))
    if alphar_>= 0
        Cr_ = -C_a*sec(alphar_)^2+C_a^2/(3*miu*Fz)*(2*sec(alphar_)^2*tan(alphar_))-C_a^3/(27*miu^2*Fz^2)*(3*tan(alphar_)^2*sec(alphar_)^2);
    else
        Cr_ = -C_a*sec(alphar_)^2-C_a^2/(3*miu*Fz)*(2*sec(alphar_)^2*tan(alphar_))-C_a^3/(27*miu^2*Fz^2)*(3*tan(alphar_)^2*sec(alphar_)^2);
    end
else
    
    %the saturation region of tire model
    Fyr_ = -miu*Fz*sign(alphar_);
    Cr_ = 0;
end

%Continuous-time model
Ac = [Cr_/(m*Vx) -lr*Cr_/(m*Vx)-Vx 0 0;
    -lr*Cr_/(Iz*Vx) lr^2*Cr_/(Iz*Vx) 0 0;
    0 1 0 0;
    1 0 Vx 0];
Bc = [1/m 0;
    lf/Iz 1/Iz;
    0 0;
    0 0];
dcc = [(Fyr_-Cr_*alphar_)/m;
    -lr*(Fyr_-Cr_*alphar_)/Iz;
    -Vx*ks;
    0];

G=[Ac Bc dcc;zeros(3,7)];
M=expm(G*Ts);
A=M(1:4,1:4);
B=M(1:4,5:6);
DK=M(1:4,7);
delta_x=A*x+B*u+DK-x;
end

== matlab function LateralControllerDIY/MATLAB Function3 ==
  data: detection input; Vx input size=1; s input; emax output; emin output
function [emax,emin] = fcn(detection,Vx,s)
if detection == 1&&s>=0
    emin = -10*ones(70,1);
    emax=   10*ones(70,1);
    if s>21.75&&s<=81.75
        k=round((s-21.75)/Vx/0.2);
        k1=k-1;
        k2=k+1;
        if k2>70
            k2=70;
        end
    elseif s<=21.75&&s>6
        k=round((s-6)/Vx/0.105);
        k1=k-2;
        k2=k+2;
    else
        k=s/Vx/0.01;
        k1=k-20;
        k2=k+20;
        if k1<=0
            k1=1;
        end
        if k2>40
            s0=(k2-40)*0.01*Vx;
            k2=40+round(s0/Vx/0.03);
        end
    end
    if k2>70
        k2=70;
    end
    if k1<1
        k1=1;
    end
    k1=round(k1);
    k2=round(k2);
    emin(k1:k2)=4*ones(k2-k1+1,1);
    emax(k1:k2)=6*ones(k2-k1+1,1);
else
    emin=-10*ones(70,1);
    emax=10*ones(70,1);
end

== matlab function LateralControllerDIY/MATLAB Function ==
  data: Vyr input; U1_out output; Yawr input; Rater input; Yr input; Fyr input; Mxr input; Vyc input; Yawc input; Ratec input; Yc input; Ulast1 input; Ulast2 input; Vx input; ks input; Useq input; U2_out output; Useq_ output; fval output; exitflag output; delta_t output; emax input; emin input
function [U1_out,U2_out,Useq_,fval,exitflag,delta_t] = fcn(Vyr,Yawr,Rater,Yr, Fyr,Mxr,Vyc,Yawc,Ratec,Yc,Ulast1,Ulast2,Vx,ks,Useq,emax,emin)
%Vyr lateral velocity, Yawr yaw angle, Rater yaw rate, Yr lateral position
%Fyr lateral force in front tyre,Mxr moment generated by longitudinal force
%'r'means reference ||  'c'means current
    if Vx<0.1
        Vx=0.001;%make sure many expressions' denominator isn't 0
    end
    lr=1.67;
    threshold=0.1022;
    miu=0.7;
    rmax=9.81*miu/Vx;
%% Initilization    
    tstart=tic;%timing on
    
    Nx=4;%number of state
    Nu=2;%number of control
    Np=60;%prediction horizon
    Nc=1;%control horizon

    %reference
    r=zeros(Nx,1);%state reference
    r(1)=Vyr;
    r(2)=Yawr;
    r(3)=Rater;
    r(4)=Yr;    
    ur1=Fyr;
    ur2=Mxr;%control reference
    
    %states
    x=zeros(Nx,1);%state reference
    x(1)=Vyc;
    x(2)=Yawc;
    x(3)=Ratec;
    x(4)=Yc;   
    
    %control
    u=zeros(Nu,1);%state reference
    u(1)=Ulast1;
    u(2)=Ulast2;
    
    %get augmented states
    kesi=zeros(Nx+Nu,1);%[X;U]
    kesi(1)=x(1)-r(1);
    kesi(2)=x(2)-r(2);
    kesi(3)=x(3)-r(3);
    kesi(4)=x(4)-r(4);
    kesi(5)=u(1)-ur1;
    kesi(6)=u(2)-ur2;
    
    Ts=0.05;%sample time
    
%% Modellng->Discretization->prediction->quadratic programming
    %Modelling&Linearization&Discretization
    steps=Np+1;
    A = zeros(Nx+Nu,Nx+Nu,steps);
    B = zeros(Nx+Nu,Nu*2,steps);
    Dc = zeros(Nx+Nu,1,steps);
    C=[1 0 0 0 0 0;0 1 0 0 0 0;0 0 1 0 0 0;0 0 0 1 0 0];
    
    for ct = 1:steps
        if ct>length(Useq)
            uk = Useq(Np,:);
        else
            uk = Useq(ct,:);
        end
        uk=uk';
        [Ad, Bd, DK, delta_x] = GetDynamics(Vx,ks,x,uk,Ts);
        A(:,:,ct)=[Ad,Bd;zeros(Nu,Nx),eye(Nu)];        
        B(:,:,ct)=[Bd zeros(4,2);eye(Nu) zeros(2,2)];
        Dc(:,:,ct)=[DK;0;0];
        x=x+delta_x;    
    end
    %construct important matrix
    %Y=PHI*kesi+THETA*delta_U+OMEGA*D
    coder.varsize('PHI',[Np*Nx,Nx+Nu]);
    coder.varsize('THETA',[Np*Nx,2*Nu]);
    coder.varsize('D',[Np*(Nx+Nu),1]);
    coder.varsize('DD',[Np*Nx,1]);
    PHI=[];
    THETA=zeros(Np*Nx,2*Nu);
    D=[];
    DD=[];
    product=eye(6);
    for j=1:Np
        product=A(:,:,j)*product;
        PHI=[PHI;C*product];
        D=[D;Dc(:,:,j)];
    end
    for k=1:Nc
        product1=eye(6);
        for j=k:Np
            THETA(4*j-3:4*j,4*k-3:4*k)=C*product1*B(:,:,Nc);
            product1=A(:,:,j+1)*product1;
        end
    end
    coder.varsize('OMEGA',[Nx*Np,(Nx+Nu)*Np]);
    OMEGA=zeros(Nx*Np,(Nx+Nu)*Np);
    for i=1:Np
        product2=A(:,:,i+1);
        for j=i:Np-1
            if i==j
                OMEGA(4*i-3:4*i,6*i-5:6*i)=C*eye(6);
            end
            OMEGA(4*j+1:4*j+4,6*j+1:6*j+6)=C*product2;
            product2=A(:,:,j+2)*product2;
        end
    end
    DD=OMEGA*D;        
    Sigma=repmat([1 0 1 0;0 1 0 1],Np,1);
    Sigma(1:2,1:4)=[1 0 0 0;0 1 0 0];
    UT=kron(ones(Np,1),[u(1);u(2)]);
    error=PHI*kesi;
    Q=kron(eye(Np,Np),diag([0 0 100 4]));    
    R=kron(eye(Np,Np),diag([0 4e-5]));    
    P=diag([3e-5 8e-5 3e-5 8e-5]);
    rou1=3e3;    
    rou2=5e4;
    H=2*[THETA'*Q*THETA+Sigma'*R*Sigma+P zeros(4,2);zeros(1,4) rou1 0;zeros(1,4) 0 rou2];%是否要乘2？要
    f=[2*(error'*Q*THETA+(OMEGA*D)'*Q*THETA+UT'*R*Sigma),0,0];%是否要转置？好像无所谓
   %% constraints
    %inequation
    A_I=[1 0 0 0;0 1 0 0;1 0 1 0;0 1 0 1]; 
    Ut=kron(ones(2,1),[Ulast1;Ulast2]);%control in last control step
    umin=[-1e4; -1e3];
    umax=[1e4; 1e3];
    Umin=kron(ones(2,1),umin);
    Umax=kron(ones(2,1),umax);
    coder.varsize('A_cons',[Np*6+8,6]);
    coder.varsize('b_cons',[Np*6+8,1]);
    A_cons=[A_I zeros(4,2);-A_I zeros(4,2)];
    b_cons=[Umax-Ut;-Umin+Ut];
    %add handling envelop constriants & environment envolop
    gamas=[1 -lr 0 0;-1 lr 0 0;0 1 0 0;0 -1 0 0];
    gamae=[0 0 0 1;0 0 0 -1];
    Gs=[Vx*threshold;Vx*threshold;rmax;rmax];
    for i=1:Np
        A_cons=[A_cons;[gamas*THETA(4*i-3:4*i,:) -ones(4,1) zeros(4,1)];[gamae*THETA(4*i-3:4*i,:) zeros(2,1) -ones(2,1)]];
        b_cons=[b_cons;[Gs-gamas*(PHI(4*i-3:4*i,:)*kesi-DD(4*i-3:4*i,:))];[emax(i);-emin(i)]-gamae*(PHI(4*i-3:4*i,:)*kesi-DD(4*i-3:4*i,:))];
    end
    
    %upper and lower boundary
    delta_umin=[-1e4;-1e3];
    delta_umax=[1e4;1e3];
    M1=10; %related to slack variable
    M2=10; %related to slack variable
    delta_Umin=kron(ones(2,1),delta_umin);
    delta_Umax=kron(ones(2,1),delta_umax);
    lb=[delta_Umin;0;0];
    ub=[delta_Umax;M1;M2];  
   %% solve quadratic programming
    opts = optimoptions('quadprog','Algorithm','active-set');
    x_start=zeros(Nu*2+2,1);%+2 corresponds to slack variables
    [X,fval,exitflag]=quadprog(H,f',A_cons,b_cons,[],[],lb,ub,x_start,opts);
    
   %% calculate control signal
    U1=kesi(5)+X(1);%The output error at the previous time plus the optimization result to get the error at this time
    U2=kesi(6)+X(2);%The output error at the previous time plus the optimization result to get the error at this time
    U1_out=U1+ur1;%Error plus reference value to get final output value    
    U2_out=U2+ur2;
    Useq_=[U1_out U2_out; repmat([U1_out+X(3) U2_out+X(4)],Np,1)];
    delta_t=toc(tstart);%timing off
end

function [A, B, DK, delta_x] = GetDynamics(Vx,ks,x,u,Ts)

%Plant Model parameters
m = 2272;   %mass
Iz = 4600;  %rotational inertia
lf = 1.11;  % distance from front axle to the mass center
lr = 1.67;  % distance from rear axle to the mass center
C_a = 1.822e5; % rear cornering stiffness 

%Enviroment parameters
miu = 0.7; %frction cooeficient 0.7 for dry road and 0.4 for wet
g = 9.81; % gravity

Fz = m*g*lf/(lf+lr); % the load that beared by the rear tire

%calculate alpha
Vy = x(1); %lateral velocity
r = x(2);  %yaw rate
alphar_ = Vy/Vx-lr*r/Vx;   %calculate linearzing point

%tire model
threshold = atan(3*miu*Fz/C_a);     % threshold for the tire linear region
if abs(alphar_)<threshold
    %the rear lateral force value (f(x0)) at the linearzing point
    Fyr_ = -C_a*tan(alphar_)+C_a^2/(3*miu*Fz)*abs(tan(alphar_))*tan(alphar_)-C_a^3/(27*miu^2*Fz^2)*tan(alphar_)^3;
    
    %the slope of linearized model (f‘(x0))
    if alphar_>= 0
        Cr_ = -C_a*sec(alphar_)^2+C_a^2/(3*miu*Fz)*(2*sec(alphar_)^2*tan(alphar_))-C_a^3/(27*miu^2*Fz^2)*(3*tan(alphar_)^2*sec(alphar_)^2);
    else
        Cr_ = -C_a*sec(alphar_)^2-C_a^2/(3*miu*Fz)*(2*sec(alphar_)^2*tan(alphar_))-C_a^3/(27*miu^2*Fz^2)*(3*tan(alphar_)^2*sec(alphar_)^2);
    end
else
    
    %the saturation region of tire model
    Fyr_ = -miu*Fz*sign(alphar_);
    Cr_ = 0;
end

%Continuous-time model
Ac = [Cr_/(m*Vx) -lr*Cr_/(m*Vx)-Vx 0 0;
    -lr*Cr_/(Iz*Vx) lr^2*Cr_/(Iz*Vx) 0 0;
    0 1 0 0;
    1 0 Vx 0];
Bc = [1/m 0;
    lf/Iz 1/Iz;
    0 0;
    0 0];
dcc = [(Fyr_-Cr_*alphar_)/m;
    -lr*(Fyr_-Cr_*alphar_)/Iz;
    -Vx*ks;
    0];

G=[Ac Bc dcc;zeros(3,7)];
M=expm(G*Ts);
A=M(1:4,1:4);
B=M(1:4,5:6);
DK=M(1:4,7);
delta_x=A*x+B*u+DK-x;
end

== matlab function LateralControllerDIY/MATLAB Function2 ==
  data: detection input; ymax output size=[PredictionHorizon,4]; Vx input size=1; x input size=[4,1]; s input; PredictionHorizon parameter; ymin output size=[PredictionHorizon,4]; Ts parameter; emax output; emin output
function [ymax, ymin, emax,emin] = fcn(detection,Vx,x,s, PredictionHorizon, Ts)

miu = 0.7; %frction cooeficient 0.7 for dry road and 0.4 for wet
g = 9.81; % gravity
m = 2272;   %mass
lf = 1.11;  % distance from front axle to the mass center
lr = 1.67;  % distance from rear axle to the mass center
C_a = 1.3e5; % rear cornering stifness

Fz = m*g*lf/(lf+lr); % the load that beared by the rear tire

rmax = g*miu/Vx; %max yaw rate
threshold = atan(3*miu*Fz/C_a);

r = x(2);
vmax = lr*r+Vx*threshold;   %max lateral velocity
vmin = lr*r-Vx*threshold;   %min lateral velocity
k = round(s/Vx/Ts);
if k>PredictionHorizon
    k =PredictionHorizon;
elseif k<20
    k=20;
end

if detection == 1
    ymin1 = [vmin -rmax -pi/2 -10];%50m is the distance from which obstacle is detected
    ymax1 = [vmax rmax pi/2 10];
    emin = -10*ones(PredictionHorizon,1);
    emax=   10*ones(PredictionHorizon,1);
    ymin = repmat(ymin1,PredictionHorizon,1);
    ymax = repmat(ymax1,PredictionHorizon,1);
    k1=k-round(3/Vx/Ts);
    k2=k+round(3/Vx/Ts);
    if k1<1
        k1=1;
    end
    if k2>PredictionHorizon
        k2=PredictionHorizon;
    end
    ymin(k1:k2,4)=4;
    ymax(k1:k2,4)=6;
    emin(k1:k2)=4;
    emax(k1:k2)=6;
else
    ymin1 = [vmin -rmax -pi/2 -10];
    ymax1 = [vmax rmax pi/2 10];
    ymin = repmat(ymin1,PredictionHorizon,1);
    ymax = repmat(ymax1,PredictionHorizon,1);
    emin=-10*ones(PredictionHorizon,1);
    emax=10*ones(PredictionHorizon,1);
end

== matlab function LateralControllerDIY/lateral dynamics1/Lateral Dynamics of plant model ==
  data: Vx input; ks input; x input; u input; xdot output; alphar_ output
function [xdot,alphar_] = fcn(Vx,ks, x, u)

%Plant Model parameters
m = 2272;   %mass
Iz = 4600;  %rotational inertia
lf = 1.11;  % distance from front axle to the mass center
lr = 1.67;  % distance from rear axle to the mass center
C_a = 1.822e5; % rear cornering stifness 

%Enviroment parameters
miu = 0.7; %frction cooeficient 0.7 for dry road and 0.4 for wet
g = 9.81; % gravity

Fz = m*g*lf/(lf+lr); % the load that beared by the rear tire

%calculate alpha
Vy = x(1); %lateral velocity
r = x(2);  %yaw rate
alphar_ = Vy/Vx-lr*r/Vx;   %calculate linearzing point

%tire model
threshold = atan(3*miu*Fz/C_a);
if abs(alphar_)<threshold
    Fyr_ = -C_a*tan(alphar_)+C_a^2/(3*miu*Fz)*abs(tan(alphar_))*tan(alphar_)-C_a^3/(27*miu^2*Fz^2)*tan(alphar_)^3;
    if alphar_>= 0
        Cr_ = -C_a*sec(alphar_)^2+C_a^2/(3*miu*Fz)*(2*sec(alphar_)^2*tan(alphar_))-C_a^3/(27*miu^2*Fz^2)*(3*tan(alphar_)^2*sec(alphar_)^2);
    else
        Cr_ = -C_a*sec(alphar_)^2-C_a^2/(3*miu*Fz)*(2*sec(alphar_)^2*tan(alphar_))-C_a^3/(27*miu^2*Fz^2)*(3*tan(alphar_)^2*sec(alphar_)^2);
    end
else
    Fyr_ = -miu*Fz*sign(alphar_);
    Cr_ = 0;
end

%Continuous-time model
Ac = [Cr_/(m*Vx) -lr*Cr_/(m*Vx)-Vx 0 0;
    -lr*Cr_/(Iz*Vx) lr^2*Cr_/(Iz*Vx) 0 0;
    0 1 0 0;
    1 0 Vx 0];
Bc = [1/m 0;
    lf/Iz 1/Iz;
    0 0;
    0 0];
dcc = [(Fyr_-Cr_*alphar_)/m;
    -lr*(Fyr_-Cr_*alphar_)/Iz;
    -Vx*ks;
    0];

% Cc =eye(4);
% Dc =zeros(4,2);
xdot = Ac*x + Bc*u +dcc;
% y = C*x + D*u;
